simulink model "PassStFtTrgtPosSelc"  (R2018b)
settings: Solver=FixedStepDiscrete  StartTime=0.0  StopTime=10.0  FixedStep=0.01  RelTol=1e-3
undefined symbols (not defined in the file or in its folder): KeSMSuSecRwStVIPFtrstRefAngle_Val, KeSMSw6sAcsEntryPassStFtUpwdDnwdPos_Val, KeSMSw6sAcsEntryPassStFtUpwdDnwdPosMiax_Val, KeSMSw6sAcsEntryPassStFtUpwdDnwdPosMin_Val, KeSMSw6sAcsExtPassStFtUpwdDnwdPos_Val, KeSMSw6sAcsExtPassStFtUpwdDnwdPosMax_Val, KeSMSw6sAcsExtPassStFtUpwdDnwdPosMin_Val, KeSMSwAcsEntryPassStFtUpwdDnwdPos_Val, KeSMSwAcsEntryPassStFtUpwdDnwdPosMiax_Val, KeSMSwAcsEntryPassStFtUpwdDnwdPosMin_Val, KeSMSwAcsExtPassStFtUpwdDnwdPos_Val, KeSMSwAcsExtPassStFtUpwdDnwdPosMax_Val, KeSMSwAcsExtPassStFtUpwdDnwdPosMin_Val
libraries: TrgtPosSelcLib x4
settings Model: ModifiedHistory=复位模式脚蹬由于没有外部标定，全都改为常量0  Creator=sn2xws  LastModifiedBy=sn2xws
settings DataIOCC: SaveFormat=StructureWithTime
settings OptimizationCC: DefaultParameterBehavior=Inlined  EnhancedBackFolding=on  PassReuseOutputArgsAs=Individual arguments  ZeroExternalMemoryAtStartup=off  ZeroInternalMemoryAtStartup=off  OptimizeBlockOrder=speed  DifferentSizesBufferReuse=on  OptimizationCustomize=off
settings DebuggingCC: ParameterTunabilityLossMsg=error
settings ModelReferenceCC: ModelReferenceNumInstancesAllowed=Single
settings SFSimCC: MATLABDynamicMemAlloc=off
settings RTWCC: SystemTargetFile=autosar.tlc  GenCodeOnly=on  TemplateMakefile=ert_default_tmf  Description=AUTOSAR  GenerateReport=on  IncludeHyperlinkInReport=on  LaunchReport=on  GenerateTraceInfo=on  GenerateTraceReport=on  GenerateTraceReportSl=on  GenerateTraceReportSf=on  GenerateTraceReportEml=on  GenerateCodeMetricsReport=on
settings CodeAppCC: ForceParamTrailComments=on  IgnoreCustomStorageClasses=off  OperatorAnnotations=on  SimulinkDataObjDesc=on  SFDataObjDesc=on  InsertBlockDesc=on
settings STFCustomTargetCC: TargetLangStandard=C99 (ISO)  MultiwordLength=256  ParMdlRefBuildCompliant=on  CompOptLevelCompliant=on  IncludeMdlTerminateFcn=off  CombineOutputUpdateFcns=on  SuppressErrorStatus=on  ERTCustomFileBanners=on  SupportNonFinite=off  SupportComplex=off  SupportContinuousTime=off  SupportNonInlinedSFcns=off  RemoveResetFunc=on  MATLABClassNameForMDSCustomization=Simulink.SoftwareTarget.ERTCustomization  AutosarCompliant=on  UseToolchainInfoCompliant=on  LookupTableObjectStructAxisOrder=2,1,3,4,...  LUTObjectStructOrderEvenSpacing=Size,Table,Breakpoints  SystemTargetFile=autosar.tlc
settings ERTTargetCC: TargetLangStandard=C99 (ISO)  ConcurrentExecutionCompliant=off  IncludeMdlTerminateFcn=off  SuppressErrorStatus=on  SupportNonFinite=off  SupportComplex=off  ModelStepFunctionPrototypeControlCompliant=off  CPPClassGenCompliant=off  AutosarCompliant=on  LookupTableObjectStructAxisOrder=2,1,3,4,...  LUTObjectStructOrderEvenSpacing=Size,Table,Breakpoints  InlinedParameterPlacement=NonHierarchical  ERTCustomFileTemplate=example_file_process.tlc  ERTFilePackagingFormat=Compact

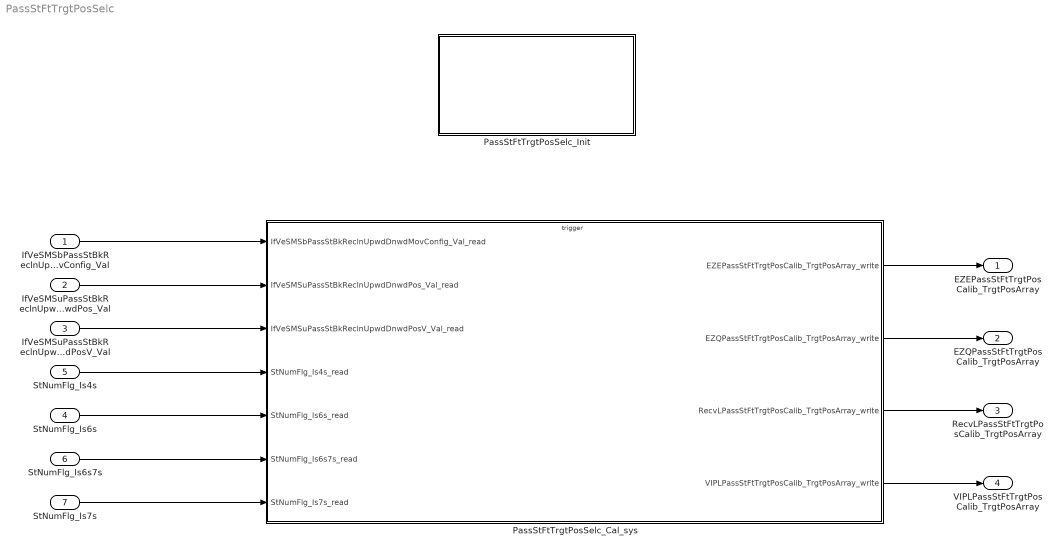
== system PassStFtTrgtPosSelc ==
  IfVeSMSbPassStBkReclnUpwdDnwdMovConfig_Val : Inport  OutDataTypeStr=boolean  PortDimensions=1
  IfVeSMSuPassStBkReclnUpwdDnwdPos_Val : Inport  Port=2  OutDataTypeStr=uint16  PortDimensions=1
  IfVeSMSuPassStBkReclnUpwdDnwdPosV_Val : Inport  Port=3  OutDataTypeStr=boolean  PortDimensions=1
  StNumFlg_Is6s : Inport  Port=4  OutDataTypeStr=boolean  PortDimensions=1
  StNumFlg_Is4s : Inport  Port=5  OutDataTypeStr=boolean  PortDimensions=1
  StNumFlg_Is6s7s : Inport  Port=6  OutDataTypeStr=boolean  PortDimensions=1
  StNumFlg_Is7s : Inport  Port=7  OutDataTypeStr=boolean  PortDimensions=1
  PassStFtTrgtPosSelc_Cal_sys : Subsystem
  PassStFtTrgtPosSelc_Init : Subsystem
  EZEPassStFtTrgtPosCalib_TrgtPosArray : Outport  Description=|  OutDataTypeStr=uint16  PortDimensions=3
      | 0:Pos
      | 1:Max
      | 2:Min
  EZQPassStFtTrgtPosCalib_TrgtPosArray : Outport  Description=|  Port=2  OutDataTypeStr=uint16  PortDimensions=3
      | 0:Pos
      | 1:Max
      | 2:Min
  RecvLPassStFtTrgtPosCalib_TrgtPosArray : Outport  Description=|  Port=3  OutDataTypeStr=uint16  PortDimensions=3
      | 0:Pos
      | 1:Max
      | 2:Min
  VIPLPassStFtTrgtPosCalib_TrgtPosArray : Outport  Description=|  Port=4  OutDataTypeStr=uint16  PortDimensions=3
      | 0:Pos
      | 1:Max
      | 2:Min
  wires:
  PassStFtTrgtPosSelc_Cal_sys/1(EZEPassStFtTrgtPosCalib_TrgtPosArray_write) -> EZEPassStFtTrgtPosCalib_TrgtPosArray/1
  PassStFtTrgtPosSelc_Cal_sys/2(EZQPassStFtTrgtPosCalib_TrgtPosArray_write) -> EZQPassStFtTrgtPosCalib_TrgtPosArray/1
  PassStFtTrgtPosSelc_Cal_sys/3(RecvLPassStFtTrgtPosCalib_TrgtPosArray_write) -> RecvLPassStFtTrgtPosCalib_TrgtPosArray/1
  PassStFtTrgtPosSelc_Cal_sys/4(VIPLPassStFtTrgtPosCalib_TrgtPosArray_write) -> VIPLPassStFtTrgtPosCalib_TrgtPosArray/1
  StNumFlg_Is6s7s/1 -> PassStFtTrgtPosSelc_Cal_sys/6(StNumFlg_Is6s7s_read)
  StNumFlg_Is7s/1 -> PassStFtTrgtPosSelc_Cal_sys/7(StNumFlg_Is7s_read)
  IfVeSMSuPassStBkReclnUpwdDnwdPosV_Val/1 -> PassStFtTrgtPosSelc_Cal_sys/3(IfVeSMSuPassStBkReclnUpwdDnwdPosV_Val_read)
  IfVeSMSuPassStBkReclnUpwdDnwdPos_Val/1 -> PassStFtTrgtPosSelc_Cal_sys/2(IfVeSMSuPassStBkReclnUpwdDnwdPos_Val_read)
  IfVeSMSbPassStBkReclnUpwdDnwdMovConfig_Val/1 -> PassStFtTrgtPosSelc_Cal_sys/1(IfVeSMSbPassStBkReclnUpwdDnwdMovConfig_Val_read)
  StNumFlg_Is4s/1 -> PassStFtTrgtPosSelc_Cal_sys/4(StNumFlg_Is4s_read)
  StNumFlg_Is6s/1 -> PassStFtTrgtPosSelc_Cal_sys/5(StNumFlg_Is6s_read)

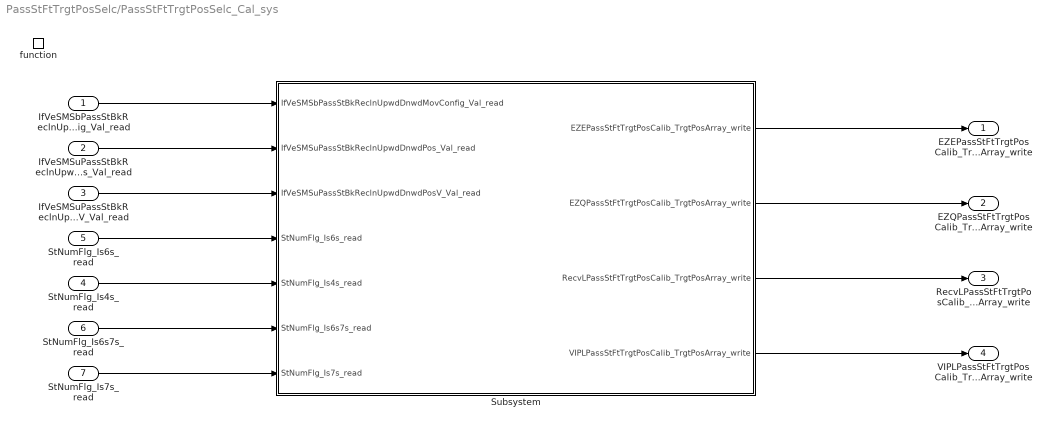
== system PassStFtTrgtPosSelc/PassStFtTrgtPosSelc_Cal_sys ==
  IfVeSMSbPassStBkReclnUpwdDnwdMovConfig_Val_read : Inport
  IfVeSMSuPassStBkReclnUpwdDnwdPos_Val_read : Inport  Port=2
  IfVeSMSuPassStBkReclnUpwdDnwdPosV_Val_read : Inport  Port=3
  StNumFlg_Is4s_read : Inport  Port=4
  StNumFlg_Is6s_read : Inport  Port=5
  StNumFlg_Is6s7s_read : Inport  Port=6
  StNumFlg_Is7s_read : Inport  Port=7
  function : TriggerPort  TriggerType=function-call  IsSimulinkFunction=on  FunctionName=PassStFtTrgtPosSelc_Cal  VariantControl=(inherit)
  Subsystem : Subsystem
  EZEPassStFtTrgtPosCalib_TrgtPosArray_write : Outport
      settings: EnsureOutportIsVirtual=on
  EZQPassStFtTrgtPosCalib_TrgtPosArray_write : Outport  Port=2
      settings: EnsureOutportIsVirtual=on
  RecvLPassStFtTrgtPosCalib_TrgtPosArray_write : Outport  Port=3
      settings: EnsureOutportIsVirtual=on
  VIPLPassStFtTrgtPosCalib_TrgtPosArray_write : Outport  Port=4
      settings: EnsureOutportIsVirtual=on
  wires:
  StNumFlg_Is4s_read/1 -> Subsystem/5(StNumFlg_Is4s_read)
  StNumFlg_Is6s7s_read/1 -> Subsystem/6(StNumFlg_Is6s7s_read)
  Subsystem/1(EZEPassStFtTrgtPosCalib_TrgtPosArray_write) -> EZEPassStFtTrgtPosCalib_TrgtPosArray_write/1
  Subsystem/2(EZQPassStFtTrgtPosCalib_TrgtPosArray_write) -> EZQPassStFtTrgtPosCalib_TrgtPosArray_write/1
  Subsystem/3(RecvLPassStFtTrgtPosCalib_TrgtPosArray_write) -> RecvLPassStFtTrgtPosCalib_TrgtPosArray_write/1
  Subsystem/4(VIPLPassStFtTrgtPosCalib_TrgtPosArray_write) -> VIPLPassStFtTrgtPosCalib_TrgtPosArray_write/1
  StNumFlg_Is6s_read/1 -> Subsystem/4(StNumFlg_Is6s_read)
  StNumFlg_Is7s_read/1 -> Subsystem/7(StNumFlg_Is7s_read)
  IfVeSMSbPassStBkReclnUpwdDnwdMovConfig_Val_read/1 -> Subsystem/1(IfVeSMSbPassStBkReclnUpwdDnwdMovConfig_Val_read)
  IfVeSMSuPassStBkReclnUpwdDnwdPos_Val_read/1 -> Subsystem/2(IfVeSMSuPassStBkReclnUpwdDnwdPos_Val_read)
  IfVeSMSuPassStBkReclnUpwdDnwdPosV_Val_read/1 -> Subsystem/3(IfVeSMSuPassStBkReclnUpwdDnwdPosV_Val_read)

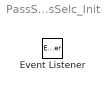
== system PassStFtTrgtPosSelc/PassStFtTrgtPosSelc_Init ==
  Event Listener : EventListener  EventName=reset

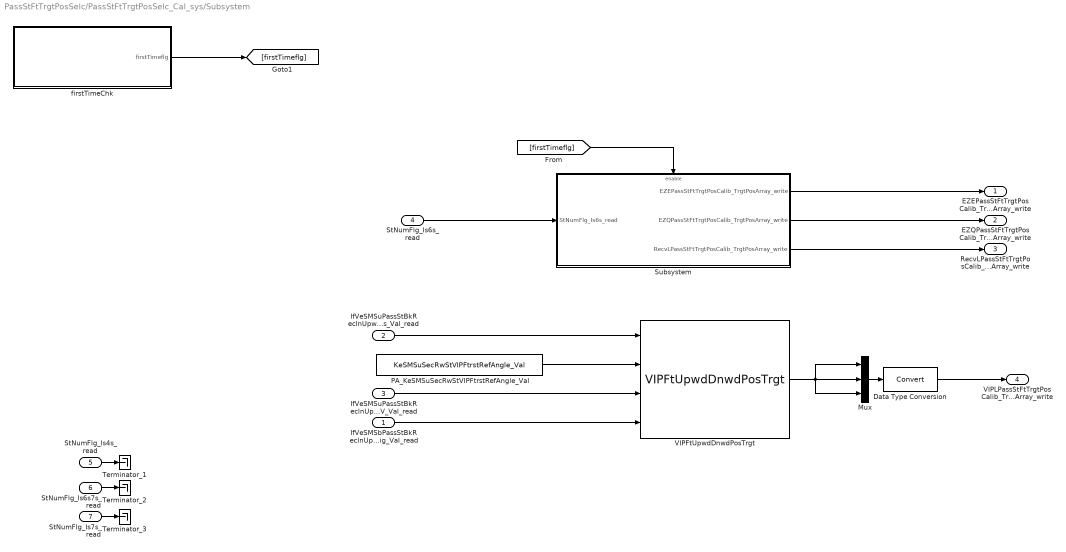
== system PassStFtTrgtPosSelc/PassStFtTrgtPosSelc_Cal_sys/Subsystem ==
  IfVeSMSbPassStBkReclnUpwdDnwdMovConfig_Val_read : Inport
  IfVeSMSuPassStBkReclnUpwdDnwdPos_Val_read : Inport  Port=2
  IfVeSMSuPassStBkReclnUpwdDnwdPosV_Val_read : Inport  Port=3
  StNumFlg_Is6s_read : Inport  Port=4
  StNumFlg_Is4s_read : Inport  Port=5
  StNumFlg_Is6s7s_read : Inport  Port=6
  StNumFlg_Is7s_read : Inport  Port=7
  Data Type Conversion : DataTypeConversion
  Mux : Mux  Inputs=3
  PA_KeSMSuSecRwStVIPFtrstRefAngle_Val : Constant  Value=KeSMSuSecRwStVIPFtrstRefAngle_Val
  Subsystem : Subsystem
  Terminator_1 : Terminator
  Terminator_2 : Terminator
  Terminator_3 : Terminator
  VIPFtUpwdDnwdPosTrgt : TrgtPosSelcLib/VIPFtUpwdDnwdPosTrgt  SystemSampleTime=-1
  firstTimeChk : Stateflow chart  TreatAsAtomicUnit=on
  EZEPassStFtTrgtPosCalib_TrgtPosArray_write : Outport
      settings: EnsureOutportIsVirtual=on
  EZQPassStFtTrgtPosCalib_TrgtPosArray_write : Outport  Port=2
      settings: EnsureOutportIsVirtual=on
  RecvLPassStFtTrgtPosCalib_TrgtPosArray_write : Outport  Port=3
      settings: EnsureOutportIsVirtual=on
  VIPLPassStFtTrgtPosCalib_TrgtPosArray_write : Outport  Port=4
      settings: EnsureOutportIsVirtual=on
  wires:
  VIPFtUpwdDnwdPosTrgt/1 -> Mux/3, Mux/1, Mux/2
  PA_KeSMSuSecRwStVIPFtrstRefAngle_Val/1 -> VIPFtUpwdDnwdPosTrgt/2
  Mux/1 -> Data Type Conversion/1
  StNumFlg_Is4s_read/1 -> Terminator_1/1
  IfVeSMSuPassStBkReclnUpwdDnwdPos_Val_read/1 -> VIPFtUpwdDnwdPosTrgt/1
  StNumFlg_Is6s7s_read/1 -> Terminator_2/1
  StNumFlg_Is7s_read/1 -> Terminator_3/1
  IfVeSMSuPassStBkReclnUpwdDnwdPosV_Val_read/1 -> VIPFtUpwdDnwdPosTrgt/3
  IfVeSMSbPassStBkReclnUpwdDnwdMovConfig_Val_read/1 -> VIPFtUpwdDnwdPosTrgt/4
  firstTimeChk/1(firstTimeflg) -> [firstTimeflg]
  StNumFlg_Is6s_read/1 -> Subsystem/1(StNumFlg_Is6s_read)
  Subsystem/1(EZEPassStFtTrgtPosCalib_TrgtPosArray_write) -> EZEPassStFtTrgtPosCalib_TrgtPosArray_write/1
  Subsystem/2(EZQPassStFtTrgtPosCalib_TrgtPosArray_write) -> EZQPassStFtTrgtPosCalib_TrgtPosArray_write/1
  Subsystem/3(RecvLPassStFtTrgtPosCalib_TrgtPosArray_write) -> RecvLPassStFtTrgtPosCalib_TrgtPosArray_write/1
  [firstTimeflg] -> Subsystem/Enable
  Data Type Conversion/1 -> VIPLPassStFtTrgtPosCalib_TrgtPosArray_write/1

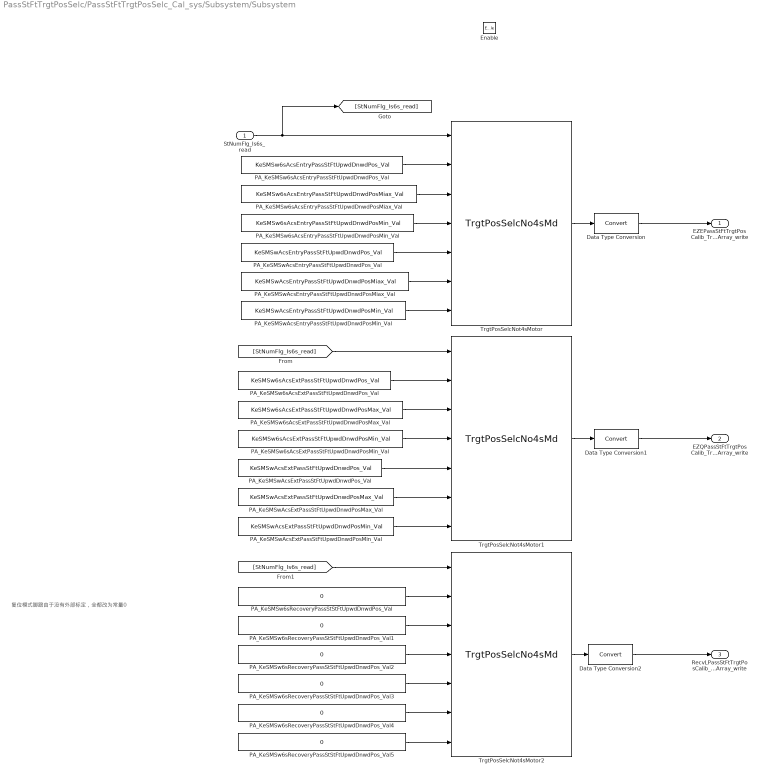
== system PassStFtTrgtPosSelc/PassStFtTrgtPosSelc_Cal_sys/Subsystem/Subsystem ==
  note: 复位模式脚蹬由于没有外部标定，全都改为常量0
  StNumFlg_Is6s_read : Inport
  Enable : EnablePort
  Data Type Conversion : DataTypeConversion
  Data Type Conversion1 : DataTypeConversion
  Data Type Conversion2 : DataTypeConversion
  PA_KeSMSw6sAcsEntryPassStFtUpwdDnwdPosMiax_Val : Constant  Value=KeSMSw6sAcsEntryPassStFtUpwdDnwdPosMiax_Val
  PA_KeSMSw6sAcsEntryPassStFtUpwdDnwdPosMin_Val : Constant  Value=KeSMSw6sAcsEntryPassStFtUpwdDnwdPosMin_Val
  PA_KeSMSw6sAcsEntryPassStFtUpwdDnwdPos_Val : Constant  Value=KeSMSw6sAcsEntryPassStFtUpwdDnwdPos_Val
  PA_KeSMSw6sAcsExtPassStFtUpwdDnwdPosMax_Val : Constant  Value=KeSMSw6sAcsExtPassStFtUpwdDnwdPosMax_Val
  PA_KeSMSw6sAcsExtPassStFtUpwdDnwdPosMin_Val : Constant  Value=KeSMSw6sAcsExtPassStFtUpwdDnwdPosMin_Val
  PA_KeSMSw6sAcsExtPassStFtUpwdDnwdPos_Val : Constant  Value=KeSMSw6sAcsExtPassStFtUpwdDnwdPos_Val
  PA_KeSMSw6sRecoveryPassStStFtUpwdDnwdPos_Val{,1..5} (6 alike) : Constant  Value=0  OutDataTypeStr=uint16
  PA_KeSMSwAcsEntryPassStFtUpwdDnwdPosMiax_Val : Constant  Value=KeSMSwAcsEntryPassStFtUpwdDnwdPosMiax_Val
  PA_KeSMSwAcsEntryPassStFtUpwdDnwdPosMin_Val : Constant  Value=KeSMSwAcsEntryPassStFtUpwdDnwdPosMin_Val
  PA_KeSMSwAcsEntryPassStFtUpwdDnwdPos_Val : Constant  Value=KeSMSwAcsEntryPassStFtUpwdDnwdPos_Val
  PA_KeSMSwAcsExtPassStFtUpwdDnwdPosMax_Val : Constant  Value=KeSMSwAcsExtPassStFtUpwdDnwdPosMax_Val
  PA_KeSMSwAcsExtPassStFtUpwdDnwdPosMin_Val : Constant  Value=KeSMSwAcsExtPassStFtUpwdDnwdPosMin_Val
  PA_KeSMSwAcsExtPassStFtUpwdDnwdPos_Val : Constant  Value=KeSMSwAcsExtPassStFtUpwdDnwdPos_Val
  TrgtPosSelcNot4sMotor : TrgtPosSelcLib/TrgtPosSelcNo4sMd  SystemSampleTime=-1
  TrgtPosSelcNot4sMotor1 : TrgtPosSelcLib/TrgtPosSelcNo4sMd  SystemSampleTime=-1
  TrgtPosSelcNot4sMotor2 : TrgtPosSelcLib/TrgtPosSelcNo4sMd  SystemSampleTime=-1
  EZEPassStFtTrgtPosCalib_TrgtPosArray_write : Outport
      settings: EnsureOutportIsVirtual=on
  EZQPassStFtTrgtPosCalib_TrgtPosArray_write : Outport  Port=2
      settings: EnsureOutportIsVirtual=on
  RecvLPassStFtTrgtPosCalib_TrgtPosArray_write : Outport  Port=3
      settings: EnsureOutportIsVirtual=on
  wires:
  PA_KeSMSwAcsExtPassStFtUpwdDnwdPos_Val/1 -> TrgtPosSelcNot4sMotor1/5
  TrgtPosSelcNot4sMotor1/1 -> Data Type Conversion1/1
  PA_KeSMSw6sAcsExtPassStFtUpwdDnwdPos_Val/1 -> TrgtPosSelcNot4sMotor1/2
  [StNumFlg_Is6s_read] -> TrgtPosSelcNot4sMotor2/1
  PA_KeSMSw6sAcsEntryPassStFtUpwdDnwdPos_Val/1 -> TrgtPosSelcNot4sMotor/2
  PA_KeSMSw6sAcsExtPassStFtUpwdDnwdPosMax_Val/1 -> TrgtPosSelcNot4sMotor1/3
  PA_KeSMSw6sRecoveryPassStStFtUpwdDnwdPos_Val/1 -> TrgtPosSelcNot4sMotor2/2
  PA_KeSMSwAcsEntryPassStFtUpwdDnwdPos_Val/1 -> TrgtPosSelcNot4sMotor/5
  [StNumFlg_Is6s_read] -> TrgtPosSelcNot4sMotor1/1
  PA_KeSMSw6sRecoveryPassStStFtUpwdDnwdPos_Val1/1 -> TrgtPosSelcNot4sMotor2/3
  PA_KeSMSw6sAcsEntryPassStFtUpwdDnwdPosMin_Val/1 -> TrgtPosSelcNot4sMotor/4
  PA_KeSMSw6sRecoveryPassStStFtUpwdDnwdPos_Val4/1 -> TrgtPosSelcNot4sMotor2/6
  PA_KeSMSwAcsEntryPassStFtUpwdDnwdPosMiax_Val/1 -> TrgtPosSelcNot4sMotor/6
  TrgtPosSelcNot4sMotor2/1 -> Data Type Conversion2/1
  PA_KeSMSwAcsExtPassStFtUpwdDnwdPosMax_Val/1 -> TrgtPosSelcNot4sMotor1/6
  PA_KeSMSwAcsExtPassStFtUpwdDnwdPosMin_Val/1 -> TrgtPosSelcNot4sMotor1/7
  PA_KeSMSw6sAcsEntryPassStFtUpwdDnwdPosMiax_Val/1 -> TrgtPosSelcNot4sMotor/3
  PA_KeSMSw6sRecoveryPassStStFtUpwdDnwdPos_Val2/1 -> TrgtPosSelcNot4sMotor2/4
  PA_KeSMSw6sRecoveryPassStStFtUpwdDnwdPos_Val3/1 -> TrgtPosSelcNot4sMotor2/5
  StNumFlg_Is6s_read/1 -> [StNumFlg_Is6s_read], TrgtPosSelcNot4sMotor/1
  PA_KeSMSw6sRecoveryPassStStFtUpwdDnwdPos_Val5/1 -> TrgtPosSelcNot4sMotor2/7
  PA_KeSMSw6sAcsExtPassStFtUpwdDnwdPosMin_Val/1 -> TrgtPosSelcNot4sMotor1/4
  TrgtPosSelcNot4sMotor/1 -> Data Type Conversion/1
  PA_KeSMSwAcsEntryPassStFtUpwdDnwdPosMin_Val/1 -> TrgtPosSelcNot4sMotor/7
  Data Type Conversion/1 -> EZEPassStFtTrgtPosCalib_TrgtPosArray_write/1
  Data Type Conversion1/1 -> EZQPassStFtTrgtPosCalib_TrgtPosArray_write/1
  Data Type Conversion2/1 -> RecvLPassStFtTrgtPosCalib_TrgtPosArray_write/1

== stateflow chart PassStFtTrgtPosSelc/PassStFtTrgtPosSelc_Cal_sys/Subsystem/firstTimeChk ==
  (default) -> (junction 1)
  (junction 1) -> (junction 5) [order 1] : [chkflg ==0]
  (junction 1) -> (junction 3) [order 2] : {firstTimeflg = 0;}
  (junction 5) -> (junction 7) : {firstTimeflg = 1;
      | chkflg=1;}
  (junction 7) -> (junction 3)
  (junction 3) -> (junction 10)
  data: chkflg local boolean size=1; firstTimeflg output boolean size=1
